simulink model "Demo_EP_IdleRandMerg"  (R2014a)
settings: Solver=FixedStepDiscrete  SolverMode=SingleTasking  StartTime=0.0  StopTime=inf  FixedStep=0.01  RelTol=1e-3
PostLoadFcn:
  | h_RPStest = RPStest;
model workspace (MAT data in the model file):
  gtest = 0
undefined symbols (not defined in the file or in its folder): avert, avert_freq_factor, avert_gaze_dirs_chance, avert_gaze_duration_factor, avert_head_frequency_factor, avert_head_speed, BML, BML1, BML2, bmlsL, bmlsM, bodyBusyFlag, clock, emotion_amount_factor, faceBusyFlag, fileID, GAZE_WIN, gazing, mut_freq_factor, mutual_gaze_duration_factor, P, pose_cat_chance, pose_chanc_factor, pose_chance_factor, pose_change_flag, pose_frequency_factor, pose_lean, pose_lean_flag, pose_speed, pose_twitch, pr, serial, STATE_BEFORE, STATE_GO, STATE_OVER, STATE_READY, Stateflow
libraries: simulink x24, instrumentlib x6, lib_affectiveChar_behavior x3, realtime_pacer_lib x2, lib_affectiveChar_input x1
(part 7 of 7)

== stateflow chart Demo_EP_IdleRandMerg/CharacterControl/custom_Behavior_Factors ==
  state setP
    entry:
    [mutual_gaze_duration_factor, avert_gaze_duration_factor,avert_head_frequency_factor,avert_head_speed,avert_gaze_dirs_chance,avert_freq_factor,mut_freq_factor]=sharedFunc.setGazeFactors(inV,inA,personality,personalityFlag,vaFlag,gazeArray);
  state init
    entry: mutual_gaze_duration_factor=1;avert_gaze_duration_factor=1;
    avert_head_frequency_factor=1;avert_head_speed=1;avert_gaze_dirs_chance=1;,avert_freq_factor=1;mut_freq_factor=1;
    pose_frequency_factor=5;pose_chanc_factor=1;pose_cat_chance=10;pose_lean=10;pose_speed=0;pose_lean_flag=0;
  state wait
  state sharedFunc [group]
  state setP1
    entry:
    [pose_twitch,pose_frequency_factor,pose_chanc_factor,pose_cat_chance,pose_lean,pose_speed,pose_lean_flag]=sharedFunc.setPoseFactors(inV,inA,personality,personalityFlag,vaFlag,poseArray,personalityChange);
  (default) -> init
  init -> wait
  setP -> wait
  wait -> setP [order 1] : [gazeArray(:,1)==1]
  setP1 -> wait
  wait -> setP1 [order 2] : [poseArray(:,1)==1]
  data: inA input double size=1; inV input double size=1; vaFlag input boolean size=1; personalityFlag input boolean size=1; gazeArray input double size=[1, 6]; personality input double size=1; personalityChange input boolean size=1; mutual_gaze_duration_factor data_store_memory; avert_head_frequency_factor data_store_memory; avert_gaze_duration_factor data_store_memory; avert_head_speed data_store_memory; avert_gaze_dirs_chance data_store_memory; poseArray input double size=[1, 6]; pose_lean data_store_memory; pose_speed data_store_memory; pose_chanc_factor data_store_memory; pose_frequency_factor data_store_memory; pose_cat_chance data_store_memory; pose_lean_flag data_store_memory; emotion_amount_custom input double size=1; emotion_amount_factor data_store_memory size=1; mut_freq_factor data_store_memory; avert_freq_factor data_store_memory; pose_twitch data_store_memory

== matlab function Demo_EP_IdleRandMerg/EmotionSubsystem/calculateValenceArousal/HELN plot ==
  data: v input; a input
function fcn(v,a)
%coder.extrinsic to bypass code generation
coder.extrinsic('fscanf')
coder.extrinsic('get_param');
% coder.extrinsic('importdata');

currentTime=get_param('Demo_EP_IdleRandMerg','SimulationTime');%use name of simulink proj

A = [v;a;currentTime];

fileID = fopen('HELN_VA_table.txt','a');
fprintf(fileID,'%0.1f,%0.1f,%0.1f\r\n',A);
fclose(fileID);

%use the following to draw the plot
%tmp_data = importdata('HEHN_VA_table.txt',','); 
%no need: x=tmp_data(:,1);y=tmp_data(:,2);z=tmp_data(:,3)
%matrix=tmp_data
%tri = delaunay(matrix(:,1),matrix(:,2));
%trisurf(tri,matrix(:,1),matrix(:,2),matrix(:,3))
%shading interp

%-----------------------------------------
% fileID = fopen('HEHN_VA_table.txt','r');
% formatSpec = '%1f\r %1f\r %1f\r\n';
% sizeA = [3 Inf];
% A = fscanf(fileID,formatSpec,sizeA)
% % A = A'
% fclose(fileID);

% x = zeros(100,2);y = zeros(100,2);
% filename = 'HEHN_VA_table.txt';
% delimiterIn = ' ';
% headerlinesIn = 1;
% A = importdata(filename,delimiterIn,headerlinesIn);

% fileID=fopen('HEHN_VA_table4.txt');
% s=textscan(fileID,'%d %d %d','headerlines',23);
% fclose(fileID);
% x=s{1}
